simulink model "rx2"  (R2022b)
settings: Solver=FixedStepDiscrete  StartTime=0.0  StopTime=3.3E6  FixedStep=1  RelTol=1e-3  EnableMultiTasking=on
model workspace (MAT data in the model file):
  mwTaskManagerKernelLatency = 0
undefined symbols (not defined in the file or in its folder): Add, jsin, magnitude, rom_pilot_conj_tt, Shift
libraries: hdlsllib x3231, whdlutilities x525, simulink x260, whdlmod x112, whdledac x26, dsphdlmathfun2 x24, commchan3 x1
(part 30 of 59)

== system rx2/process4/decoder/rate recover/Subsystem ==
  start : Inport
  Compare To Constant : simulink/Logic and Bit Operations/Compare To Constant  relop===  const=valid_length  OutDataTypeStr=boolean
  Data Type Conversion : DataTypeConversion  OutDataTypeStr=boolean  SaturateOnIntegerOverflow=off  RndMeth=Floor
  Delay1 : Delay  InitialCondition=0
  Delay2 : Delay  DelayLength=1  InitialCondition=0
  Detect Fall Nonpositive : simulink/Logic and Bit Operations/Detect Fall Nonpositive  vinit=0  OutDataTypeStr=boolean
  HDL Counter1 : hdlsllib/Sources/HDL Counter  CountType=Count limited  CountInit=1  CountStep=1  CountMax=valid_length  CountFromType=Initial value  CountFrom=1  CountResetPort=off  CountLoadPort=off  CountEnbPort=on  CountDirPort=off  CountHitOutputPort=off  CountDataType=Unsigned  CountWordLen=16  CountFracLen=0  CountSampTime=1
  HDL Counter4 : hdlsllib/Sources/HDL Counter  CountType=Count limited  CountInit=0  CountStep=1  CountMax=1  CountFromType=Initial value  CountFrom=0  CountResetPort=on  CountLoadPort=off  CountEnbPort=on  CountDirPort=off  CountHitOutputPort=off  CountDataType=Unsigned  CountWordLen=8  CountFracLen=0  CountSampTime=1
  Logical Operator4 : Logic  AllPortsSameDT=off  OutDataTypeStr=boolean
  valid_out : Outport
  start_out : Outport  Port=2
  end_out : Outport  Port=3
  wires:
  Logical Operator4/1 -> end_out/1  "end_out"
  Delay2/1 -> valid_out/1, Logical Operator4/2  "valid_out"
  Delay1/1 -> start_out/1  "start_out"
  Data Type Conversion/1 -> HDL Counter1/1, Detect Fall Nonpositive/1, Delay2/1
  Detect Fall Nonpositive/1 -> Logical Operator4/1  "symbol_end"
  start/1 -> HDL Counter4/2, Delay1/1
  HDL Counter4/1 -> Data Type Conversion/1
  HDL Counter1/1 -> Compare To Constant/1  "count_1"
  Compare To Constant/1 -> HDL Counter4/1

== system rx2/process4/decoder/s-p/S-P ==
  data_in : Inport  OutDataTypeStr=fixdt(1,16,9)
  valid_in : Inport  Port=2  OutDataTypeStr=boolean
  Deserializer1D : hdlsllib/HDL Operations/Deserializer1D  Ratio=data_len  IdleCycles=8  InitialCondition=0  startIn=off  validIn=on  validOut=on  inputDataDimensions=-1  inputSampleTime=1  inputSignalType=real
  Rate Transition : RateTransition  OutPortSampleTimeOpt=Multiple of input port sample time  OutPortSampleTimeMultiple=1/72
  Rate Transition1 : RateTransition  OutPortSampleTimeOpt=Multiple of input port sample time  OutPortSampleTimeMultiple=1/72
  data_out : Outport  OutDataTypeStr=fixdt(1,16,9)
  valid_out : Outport  Port=2  OutDataTypeStr=boolean
  wires:
  valid_in/1 -> Deserializer1D/2  "valid_in"
  Rate Transition1/1 -> valid_out/1  "valid"
  Deserializer1D/2 -> Rate Transition1/1
  Rate Transition/1 -> data_out/1  "data"
  data_in/1 -> Deserializer1D/1
  Deserializer1D/1 -> Rate Transition/1

== system rx2/process4/decoder/s-p/S-P2 ==
  data_in : Inport  OutDataTypeStr=fixdt(1,16,9)
  valid_in : Inport  Port=2  OutDataTypeStr=boolean
  Deserializer1D : hdlsllib/HDL Operations/Deserializer1D  Ratio=data_len  IdleCycles=64  InitialCondition=0  startIn=off  validIn=on  validOut=on  inputDataDimensions=-1  inputSampleTime=1  inputSignalType=real
  Rate Transition : RateTransition  OutPortSampleTimeOpt=Multiple of input port sample time  OutPortSampleTimeMultiple=1/72
  Rate Transition1 : RateTransition  OutPortSampleTimeOpt=Multiple of input port sample time  OutPortSampleTimeMultiple=1/72
  data_out : Outport  OutDataTypeStr=fixdt(1,16,9)
  valid_out : Outport  Port=2  OutDataTypeStr=boolean
  wires:
  valid_in/1 -> Deserializer1D/2  "valid_in"
  Rate Transition1/1 -> valid_out/1  "valid"
  Deserializer1D/2 -> Rate Transition1/1
  Rate Transition/1 -> data_out/1  "data"
  data_in/1 -> Deserializer1D/1
  Deserializer1D/1 -> Rate Transition/1

== system rx2/process4/decoder/soft demodule/Subsystem ==
  start : Inport
  Compare To Constant : simulink/Logic and Bit Operations/Compare To Constant  relop===  const=valid_length  OutDataTypeStr=boolean
  Data Type Conversion : DataTypeConversion  OutDataTypeStr=boolean  SaturateOnIntegerOverflow=off  RndMeth=Floor
  Delay1 : Delay  InitialCondition=0
  Delay2 : Delay  DelayLength=1  InitialCondition=0
  Detect Fall Nonpositive : simulink/Logic and Bit Operations/Detect Fall Nonpositive  vinit=0  OutDataTypeStr=boolean
  HDL Counter1 : hdlsllib/Sources/HDL Counter  CountType=Count limited  CountInit=1  CountStep=1  CountMax=valid_length  CountFromType=Initial value  CountFrom=1  CountResetPort=off  CountLoadPort=off  CountEnbPort=on  CountDirPort=off  CountHitOutputPort=off  CountDataType=Unsigned  CountWordLen=16  CountFracLen=0  CountSampTime=1
  HDL Counter4 : hdlsllib/Sources/HDL Counter  CountType=Count limited  CountInit=0  CountStep=1  CountMax=1  CountFromType=Initial value  CountFrom=0  CountResetPort=on  CountLoadPort=off  CountEnbPort=on  CountDirPort=off  CountHitOutputPort=off  CountDataType=Unsigned  CountWordLen=8  CountFracLen=0  CountSampTime=1
  Logical Operator4 : Logic  AllPortsSameDT=off  OutDataTypeStr=boolean
  valid_out : Outport
  start_out : Outport  Port=2
  end_out : Outport  Port=3
  wires:
  Logical Operator4/1 -> end_out/1  "end_out"
  Delay2/1 -> valid_out/1, Logical Operator4/2  "valid_out"
  Delay1/1 -> start_out/1  "start_out"
  Data Type Conversion/1 -> HDL Counter1/1, Detect Fall Nonpositive/1, Delay2/1
  Detect Fall Nonpositive/1 -> Logical Operator4/1  "symbol_end"
  start/1 -> HDL Counter4/2, Delay1/1
  HDL Counter4/1 -> Data Type Conversion/1
  HDL Counter1/1 -> Compare To Constant/1  "count_1"
  Compare To Constant/1 -> HDL Counter4/1

== system rx2/process4/decoder/synchronization/data_synchronization1 ==
  port1 : Inport
  port2 : Inport  Port=2
  port1_ctrl : Inport  Port=3  OutDataTypeStr=Bus: samplecontrol
  port2_ctrl : Inport  Port=4  OutDataTypeStr=Bus: samplecontrol
  Bit Concat : hdlsllib/Logic and Bit Operations/Bit Concat  numInputs=2
  Compare To Constant10 : hdlsllib/Logic and Bit Operations/Compare To Constant  relop===  const=1  OutDataTypeStr=boolean
  Constant3 : Constant  OutDataTypeStr=fixdt(0,2,0)
  Data Type Conversion1 : DataTypeConversion  OutDataTypeStr=boolean  SaturateOnIntegerOverflow=off  RndMeth=Floor
  Delay1 : Delay  DelayLength=3  InitialCondition=0  SampleTime=1
  Delay{3..7,10..11} (7 alike) : Delay  DelayLength=1  InitialCondition=0
  Delay2 : Delay  DelayLength=3  InitialCondition=0  SampleTime=1
  Delay8 : Delay  DelayLength=3  InitialCondition=0
  Delay9 : Delay  DelayLength=3  InitialCondition=0
  Detect Rise Positive : simulink/Logic and Bit Operations/Detect Rise Positive  vinit=0  OutDataTypeStr=boolean
  Detect Rise Positive5 : hdlsllib/Logic and Bit Operations/Detect Rise Positive  vinit=0  OutDataTypeStr=boolean
  Ground3 : Ground
  Ground4 : Ground
  HDL Counter3 : hdlsllib/Sources/HDL Counter  CountType=Count limited  CountInit=0  CountStep=1  CountMax=2  CountFromType=Initial value  CountFrom=0  CountResetPort=on  CountLoadPort=off  CountEnbPort=on  CountDirPort=off  CountHitOutputPort=on  CountDataType=Unsigned  CountWordLen=2  CountFracLen=0  CountSampTime=1
  HDL Counter4 : hdlsllib/Sources/HDL Counter  CountType=Count limited  CountInit=0  CountStep=1  CountMax=2  CountFromType=Initial value  CountFrom=0  CountResetPort=on  CountLoadPort=off  CountEnbPort=on  CountDirPort=off  CountHitOutputPort=on  CountDataType=Unsigned  CountWordLen=2  CountFracLen=0  CountSampTime=1
  HDL Counter5 : hdlsllib/Sources/HDL Counter  CountType=Count limited  CountInit=0  CountStep=1  CountMax=1  CountFromType=Initial value  CountFrom=0  CountResetPort=off  CountLoadPort=off  CountEnbPort=on  CountDirPort=off  CountHitOutputPort=off  CountDataType=Unsigned  CountWordLen=1  CountFracLen=0  CountSampTime=1
  HDL FIFO : hdlsllib/HDL RAMs/HDL FIFO  fifo_size=792  mode=Classic  ratio=1  push_msg=Warning  pop_msg=Ignore  show_empty=on  show_full=on  show_num=on  LabelModeActiveChoice_Mode=Classic  rst_port=off
  Logical Operator : Logic  Operator=OR  AllPortsSameDT=off  OutDataTypeStr=boolean
  Logical Operator8 : Logic  Operator=OR  AllPortsSameDT=off  OutDataTypeStr=boolean
  Logical Operator9 : Logic  Operator=OR  AllPortsSameDT=off  OutDataTypeStr=boolean
  Multiport Switch{1..5} (5 alike) : MultiPortSwitch  Inputs=2  DiagnosticForDefault=None  SaturateOnIntegerOverflow=off  InputSameDT=off
  Sample Control Bus Selector : whdlutilities/Sample Control Bus Selector  OutputSignals=start,end,valid
  Sample Control Bus Selector1 : whdlutilities/Sample Control Bus Selector  OutputSignals=start,end,valid
  Simple Dual Port RAM : hdlsllib/HDL RAMs/Simple Dual Port RAM  ram_size=2
  Switch5 : Switch  Criteria=u2 ~= 0  SaturateOnIntegerOverflow=off  InputSameDT=off
  Switch6 : Switch  Criteria=u2 ~= 0  SaturateOnIntegerOverflow=off  InputSameDT=off
  Terminator{,1..3} (4 alike) : Terminator
  port1_syn : Outport  VectorParamsAs1DForOutWhenUnconnected=off
  port2_syn : Outport  Port=2  VectorParamsAs1DForOutWhenUnconnected=off
  valid_syn : Outport  Port=3  OutDataTypeStr=boolean  VectorParamsAs1DForOutWhenUnconnected=off
  start_syn : Outport  Port=4  OutDataTypeStr=boolean  VectorParamsAs1DForOutWhenUnconnected=off
  wires:
  port1_ctrl/1 -> Sample Control Bus Selector/1
  port2_ctrl/1 -> Sample Control Bus Selector1/1
  Sample Control Bus Selector/1 -> Logical Operator/1
  Sample Control Bus Selector1/1 -> Logical Operator/2
  Sample Control Bus Selector/2 -> Logical Operator8/1
  Delay7/1 -> HDL Counter4/1
  HDL Counter4/2 -> Delay7/1
  Compare To Constant10/1 -> Detect Rise Positive5/1
  Logical Operator8/1 -> HDL Counter3/2
  HDL Counter3/2 -> Logical Operator9/2, Delay6/1
  HDL Counter3/1 -> Terminator2/1
  Delay6/1 -> HDL Counter3/1
  Logical Operator/1 -> HDL Counter4/2
  Detect Rise Positive5/1 -> Logical Operator9/1
  HDL Counter4/1 -> Compare To Constant10/1
  HDL Counter5/1 -> Data Type Conversion1/1
  Logical Operator9/1 -> HDL Counter5/1, Simple Dual Port RAM/3
  Bit Concat/1 -> Simple Dual Port RAM/1
  Constant3/1 -> Simple Dual Port RAM/4, Simple Dual Port RAM/2
  Data Type Conversion1/1 -> Delay3/1
  Sample Control Bus Selector1/2 -> Logical Operator8/2
  Simple Dual Port RAM/1 -> [number]
  port1/1 -> Delay1/1
  port2/1 -> Delay2/1
  Multiport Switch1/1 -> HDL FIFO/2
  HDL FIFO/1 -> Multiport Switch5/3, Multiport Switch4/2
  HDL FIFO/3 -> Terminator/1
  Multiport Switch3/1 -> HDL FIFO/1
  Multiport Switch2/1 -> Delay11/1, HDL FIFO/3
  [number] -> Multiport Switch2/1, Multiport Switch1/1, Multiport Switch3/1
  Sample Control Bus Selector/3 -> Delay9/1, Bit Concat/2
  Sample Control Bus Selector1/3 -> Delay8/1, Bit Concat/1
  Delay2/1 -> [P2], Multiport Switch3/3
  Delay3/1 -> [number_valid]
  Delay8/1 -> Multiport Switch2/2, Multiport Switch1/3
  Delay9/1 -> Multiport Switch2/3, Multiport Switch1/2
  HDL FIFO/2 -> Terminator1/1
  HDL FIFO/4 -> Terminator3/1
  [number] -> Delay4/1
  Delay4/1 -> Multiport Switch5/1, Multiport Switch4/1
  Delay1/1 -> [P1], Multiport Switch3/2
  [P1] -> Delay5/1
  [P2] -> Delay10/1
  Delay10/1 -> Multiport Switch5/2
  Delay5/1 -> Multiport Switch4/3
  Ground4/1 -> Switch6/3
  Switch5/1 -> port1_syn/1  "port1_syn"
  Switch6/1 -> port2_syn/1  "port2_syn"
  Ground3/1 -> Switch5/3
  Multiport Switch4/1 -> Switch5/1
  Multiport Switch5/1 -> Switch6/1
  Delay11/1 -> Switch5/2, Switch6/2, Detect Rise Positive/1, valid_syn/1
  Detect Rise Positive/1 -> start_syn/1

== system rx2/process4/decoder/synchronization/data_synchronization2 ==
  port1 : Inport
  port2 : Inport  Port=2
  port1_ctrl : Inport  Port=3  OutDataTypeStr=Bus: samplecontrol
  port2_ctrl : Inport  Port=4  OutDataTypeStr=Bus: samplecontrol
  Bit Concat : hdlsllib/Logic and Bit Operations/Bit Concat  numInputs=2
  Compare To Constant10 : hdlsllib/Logic and Bit Operations/Compare To Constant  relop===  const=1  OutDataTypeStr=boolean
  Constant3 : Constant  OutDataTypeStr=fixdt(0,2,0)
  Data Type Conversion1 : DataTypeConversion  OutDataTypeStr=boolean  SaturateOnIntegerOverflow=off  RndMeth=Floor
  Delay1 : Delay  DelayLength=3  InitialCondition=0  SampleTime=1
  Delay{3..7,10..11} (7 alike) : Delay  DelayLength=1  InitialCondition=0
  Delay2 : Delay  DelayLength=3  InitialCondition=0  SampleTime=1
  Delay8 : Delay  DelayLength=3  InitialCondition=0
  Delay9 : Delay  DelayLength=3  InitialCondition=0
  Detect Rise Positive : simulink/Logic and Bit Operations/Detect Rise Positive  vinit=0  OutDataTypeStr=boolean
  Detect Rise Positive5 : hdlsllib/Logic and Bit Operations/Detect Rise Positive  vinit=0  OutDataTypeStr=boolean
  Ground3 : Ground
  Ground4 : Ground
  HDL Counter3 : hdlsllib/Sources/HDL Counter  CountType=Count limited  CountInit=0  CountStep=1  CountMax=2  CountFromType=Initial value  CountFrom=0  CountResetPort=on  CountLoadPort=off  CountEnbPort=on  CountDirPort=off  CountHitOutputPort=on  CountDataType=Unsigned  CountWordLen=2  CountFracLen=0  CountSampTime=1
  HDL Counter4 : hdlsllib/Sources/HDL Counter  CountType=Count limited  CountInit=0  CountStep=1  CountMax=2  CountFromType=Initial value  CountFrom=0  CountResetPort=on  CountLoadPort=off  CountEnbPort=on  CountDirPort=off  CountHitOutputPort=on  CountDataType=Unsigned  CountWordLen=2  CountFracLen=0  CountSampTime=1
  HDL Counter5 : hdlsllib/Sources/HDL Counter  CountType=Count limited  CountInit=0  CountStep=1  CountMax=1  CountFromType=Initial value  CountFrom=0  CountResetPort=off  CountLoadPort=off  CountEnbPort=on  CountDirPort=off  CountHitOutputPort=off  CountDataType=Unsigned  CountWordLen=1  CountFracLen=0  CountSampTime=1
  HDL FIFO : hdlsllib/HDL RAMs/HDL FIFO  fifo_size=792  mode=Classic  ratio=1  push_msg=Warning  pop_msg=Ignore  show_empty=on  show_full=on  show_num=on  LabelModeActiveChoice_Mode=Classic  rst_port=off
  Logical Operator : Logic  Operator=OR  AllPortsSameDT=off  OutDataTypeStr=boolean
  Logical Operator8 : Logic  Operator=OR  AllPortsSameDT=off  OutDataTypeStr=boolean
  Logical Operator9 : Logic  Operator=OR  AllPortsSameDT=off  OutDataTypeStr=boolean
  Multiport Switch{1..5} (5 alike) : MultiPortSwitch  Inputs=2  DiagnosticForDefault=None  SaturateOnIntegerOverflow=off  InputSameDT=off
  Sample Control Bus Selector : whdlutilities/Sample Control Bus Selector  OutputSignals=start,end,valid
  Sample Control Bus Selector1 : whdlutilities/Sample Control Bus Selector  OutputSignals=start,end,valid
  Simple Dual Port RAM : hdlsllib/HDL RAMs/Simple Dual Port RAM  ram_size=2
  Switch5 : Switch  Criteria=u2 ~= 0  SaturateOnIntegerOverflow=off  InputSameDT=off
  Switch6 : Switch  Criteria=u2 ~= 0  SaturateOnIntegerOverflow=off  InputSameDT=off
  Terminator{,1..3} (4 alike) : Terminator
  port1_syn : Outport  VectorParamsAs1DForOutWhenUnconnected=off
  port2_syn : Outport  Port=2  VectorParamsAs1DForOutWhenUnconnected=off
  valid_syn : Outport  Port=3  OutDataTypeStr=boolean  VectorParamsAs1DForOutWhenUnconnected=off
  start_syn : Outport  Port=4  OutDataTypeStr=boolean  VectorParamsAs1DForOutWhenUnconnected=off
  wires:
  port1_ctrl/1 -> Sample Control Bus Selector/1
  port2_ctrl/1 -> Sample Control Bus Selector1/1
  Sample Control Bus Selector/1 -> Logical Operator/1
  Sample Control Bus Selector1/1 -> Logical Operator/2
  Sample Control Bus Selector/2 -> Logical Operator8/1
  Delay7/1 -> HDL Counter4/1
  HDL Counter4/2 -> Delay7/1
  Compare To Constant10/1 -> Detect Rise Positive5/1
  Logical Operator8/1 -> HDL Counter3/2
  HDL Counter3/2 -> Logical Operator9/2, Delay6/1
  HDL Counter3/1 -> Terminator2/1
  Delay6/1 -> HDL Counter3/1
  Logical Operator/1 -> HDL Counter4/2
  Detect Rise Positive5/1 -> Logical Operator9/1
  HDL Counter4/1 -> Compare To Constant10/1
  HDL Counter5/1 -> Data Type Conversion1/1
  Logical Operator9/1 -> HDL Counter5/1, Simple Dual Port RAM/3
  Bit Concat/1 -> Simple Dual Port RAM/1
  Constant3/1 -> Simple Dual Port RAM/4, Simple Dual Port RAM/2
  Data Type Conversion1/1 -> Delay3/1
  Sample Control Bus Selector1/2 -> Logical Operator8/2
  Simple Dual Port RAM/1 -> [number]
  port1/1 -> Delay1/1
  port2/1 -> Delay2/1
  Multiport Switch1/1 -> HDL FIFO/2
  HDL FIFO/1 -> Multiport Switch5/3, Multiport Switch4/2
  HDL FIFO/3 -> Terminator/1
  Multiport Switch3/1 -> HDL FIFO/1
  Multiport Switch2/1 -> HDL FIFO/3, Delay11/1
  [number] -> Multiport Switch2/1, Multiport Switch1/1, Multiport Switch3/1
  Sample Control Bus Selector/3 -> Delay9/1, Bit Concat/2
  Sample Control Bus Selector1/3 -> Delay8/1, Bit Concat/1
  Delay2/1 -> [P2], Multiport Switch3/3
  Delay3/1 -> [number_valid]
  Delay8/1 -> Multiport Switch2/2, Multiport Switch1/3
  Delay9/1 -> Multiport Switch2/3, Multiport Switch1/2
  HDL FIFO/2 -> Terminator1/1
  HDL FIFO/4 -> Terminator3/1
  [number] -> Delay4/1
  Delay4/1 -> Multiport Switch5/1, Multiport Switch4/1
  Delay1/1 -> [P1], Multiport Switch3/2
  [P1] -> Delay5/1
  [P2] -> Delay10/1
  Delay10/1 -> Multiport Switch5/2
  Delay5/1 -> Multiport Switch4/3
  Ground4/1 -> Switch6/3
  Switch5/1 -> port1_syn/1  "port1_syn"
  Switch6/1 -> port2_syn/1  "port2_syn"
  Ground3/1 -> Switch5/3
  Multiport Switch4/1 -> Switch5/1
  Multiport Switch5/1 -> Switch6/1
  Delay11/1 -> Switch5/2, Switch6/2, Detect Rise Positive/1, valid_syn/1
  Detect Rise Positive/1 -> start_syn/1

== system rx2/process4/decoder/synchronization/data_synchronization3 ==
  port1 : Inport
  port2 : Inport  Port=2
  port1_ctrl : Inport  Port=3  OutDataTypeStr=Bus: samplecontrol
  port2_ctrl : Inport  Port=4  OutDataTypeStr=Bus: samplecontrol
  Bit Concat : hdlsllib/Logic and Bit Operations/Bit Concat  numInputs=2
  Compare To Constant10 : hdlsllib/Logic and Bit Operations/Compare To Constant  relop===  const=1  OutDataTypeStr=boolean
  Constant3 : Constant  OutDataTypeStr=fixdt(0,2,0)
  Data Type Conversion1 : DataTypeConversion  OutDataTypeStr=boolean  SaturateOnIntegerOverflow=off  RndMeth=Floor
  Delay1 : Delay  DelayLength=3  InitialCondition=0  SampleTime=1
  Delay{3..7,10..11} (7 alike) : Delay  DelayLength=1  InitialCondition=0
  Delay2 : Delay  DelayLength=3  InitialCondition=0  SampleTime=1
  Delay8 : Delay  DelayLength=3  InitialCondition=0
  Delay9 : Delay  DelayLength=3  InitialCondition=0
  Detect Rise Positive : simulink/Logic and Bit Operations/Detect Rise Positive  vinit=0  OutDataTypeStr=boolean
  Detect Rise Positive5 : hdlsllib/Logic and Bit Operations/Detect Rise Positive  vinit=0  OutDataTypeStr=boolean
  Ground3 : Ground
  Ground4 : Ground
  HDL Counter3 : hdlsllib/Sources/HDL Counter  CountType=Count limited  CountInit=0  CountStep=1  CountMax=2  CountFromType=Initial value  CountFrom=0  CountResetPort=on  CountLoadPort=off  CountEnbPort=on  CountDirPort=off  CountHitOutputPort=on  CountDataType=Unsigned  CountWordLen=2  CountFracLen=0  CountSampTime=1
  HDL Counter4 : hdlsllib/Sources/HDL Counter  CountType=Count limited  CountInit=0  CountStep=1  CountMax=2  CountFromType=Initial value  CountFrom=0  CountResetPort=on  CountLoadPort=off  CountEnbPort=on  CountDirPort=off  CountHitOutputPort=on  CountDataType=Unsigned  CountWordLen=2  CountFracLen=0  CountSampTime=1
  HDL Counter5 : hdlsllib/Sources/HDL Counter  CountType=Count limited  CountInit=0  CountStep=1  CountMax=1  CountFromType=Initial value  CountFrom=0  CountResetPort=off  CountLoadPort=off  CountEnbPort=on  CountDirPort=off  CountHitOutputPort=off  CountDataType=Unsigned  CountWordLen=1  CountFracLen=0  CountSampTime=1
  HDL FIFO : hdlsllib/HDL RAMs/HDL FIFO  fifo_size=792  mode=Classic  ratio=1  push_msg=Warning  pop_msg=Ignore  show_empty=on  show_full=on  show_num=on  LabelModeActiveChoice_Mode=Classic  rst_port=off
  Logical Operator : Logic  Operator=OR  AllPortsSameDT=off  OutDataTypeStr=boolean
  Logical Operator8 : Logic  Operator=OR  AllPortsSameDT=off  OutDataTypeStr=boolean
  Logical Operator9 : Logic  Operator=OR  AllPortsSameDT=off  OutDataTypeStr=boolean
  Multiport Switch{1..5} (5 alike) : MultiPortSwitch  Inputs=2  DiagnosticForDefault=None  SaturateOnIntegerOverflow=off  InputSameDT=off
  Sample Control Bus Selector : whdlutilities/Sample Control Bus Selector  OutputSignals=start,end,valid
  Sample Control Bus Selector1 : whdlutilities/Sample Control Bus Selector  OutputSignals=start,end,valid
  Simple Dual Port RAM : hdlsllib/HDL RAMs/Simple Dual Port RAM  ram_size=2
  Switch5 : Switch  Criteria=u2 ~= 0  SaturateOnIntegerOverflow=off  InputSameDT=off
  Switch6 : Switch  Criteria=u2 ~= 0  SaturateOnIntegerOverflow=off  InputSameDT=off
  Terminator{,1..3} (4 alike) : Terminator
  port1_syn : Outport  VectorParamsAs1DForOutWhenUnconnected=off
  port2_syn : Outport  Port=2  VectorParamsAs1DForOutWhenUnconnected=off
  valid_syn : Outport  Port=3  OutDataTypeStr=boolean  VectorParamsAs1DForOutWhenUnconnected=off
  start_syn : Outport  Port=4  OutDataTypeStr=boolean  VectorParamsAs1DForOutWhenUnconnected=off
  wires:
  port1_ctrl/1 -> Sample Control Bus Selector/1
  port2_ctrl/1 -> Sample Control Bus Selector1/1
  Sample Control Bus Selector/1 -> Logical Operator/1
  Sample Control Bus Selector1/1 -> Logical Operator/2
  Sample Control Bus Selector/2 -> Logical Operator8/1
  Delay7/1 -> HDL Counter4/1
  HDL Counter4/2 -> Delay7/1
  Compare To Constant10/1 -> Detect Rise Positive5/1
  Logical Operator8/1 -> HDL Counter3/2
  HDL Counter3/2 -> Logical Operator9/2, Delay6/1
  HDL Counter3/1 -> Terminator2/1
  Delay6/1 -> HDL Counter3/1
  Logical Operator/1 -> HDL Counter4/2
  Detect Rise Positive5/1 -> Logical Operator9/1
  HDL Counter4/1 -> Compare To Constant10/1
  HDL Counter5/1 -> Data Type Conversion1/1
  Logical Operator9/1 -> HDL Counter5/1, Simple Dual Port RAM/3
  Bit Concat/1 -> Simple Dual Port RAM/1
  Constant3/1 -> Simple Dual Port RAM/4, Simple Dual Port RAM/2
  Data Type Conversion1/1 -> Delay3/1
  Sample Control Bus Selector1/2 -> Logical Operator8/2
  Simple Dual Port RAM/1 -> [number]
  port1/1 -> Delay1/1
  port2/1 -> Delay2/1
  Multiport Switch1/1 -> HDL FIFO/2
  HDL FIFO/1 -> Multiport Switch5/3, Multiport Switch4/2
  HDL FIFO/3 -> Terminator/1
  Multiport Switch3/1 -> HDL FIFO/1
  Multiport Switch2/1 -> HDL FIFO/3, Delay11/1
  [number] -> Multiport Switch2/1, Multiport Switch1/1, Multiport Switch3/1
  Sample Control Bus Selector/3 -> Delay9/1, Bit Concat/2
  Sample Control Bus Selector1/3 -> Delay8/1, Bit Concat/1
  Delay2/1 -> [P2], Multiport Switch3/3
  Delay3/1 -> [number_valid]
  Delay8/1 -> Multiport Switch2/2, Multiport Switch1/3
  Delay9/1 -> Multiport Switch2/3, Multiport Switch1/2
  HDL FIFO/2 -> Terminator1/1
  HDL FIFO/4 -> Terminator3/1
  [number] -> Delay4/1
  Delay4/1 -> Multiport Switch5/1, Multiport Switch4/1
  Delay1/1 -> [P1], Multiport Switch3/2
  [P1] -> Delay5/1
  [P2] -> Delay10/1
  Delay10/1 -> Multiport Switch5/2
  Delay5/1 -> Multiport Switch4/3
  Ground4/1 -> Switch6/3
  Switch5/1 -> port1_syn/1  "port1_syn"
  Switch6/1 -> port2_syn/1  "port2_syn"
  Ground3/1 -> Switch5/3
  Multiport Switch4/1 -> Switch5/1
  Multiport Switch5/1 -> Switch6/1
  Delay11/1 -> Switch5/2, Switch6/2, Detect Rise Positive/1, valid_syn/1
  Detect Rise Positive/1 -> start_syn/1

== system rx2/process4/decoder/synchronization/data_synchronization4 ==
  port1 : Inport
  port2 : Inport  Port=2
  port1_ctrl : Inport  Port=3  OutDataTypeStr=Bus: samplecontrol
  port2_ctrl : Inport  Port=4  OutDataTypeStr=Bus: samplecontrol
  Bit Concat : hdlsllib/Logic and Bit Operations/Bit Concat  numInputs=2
  Compare To Constant10 : hdlsllib/Logic and Bit Operations/Compare To Constant  relop===  const=1  OutDataTypeStr=boolean
  Constant3 : Constant  OutDataTypeStr=fixdt(0,2,0)
  Data Type Conversion1 : DataTypeConversion  OutDataTypeStr=boolean  SaturateOnIntegerOverflow=off  RndMeth=Floor
  Delay1 : Delay  DelayLength=3  InitialCondition=0  SampleTime=1
  Delay{3..7,10..11} (7 alike) : Delay  DelayLength=1  InitialCondition=0
  Delay2 : Delay  DelayLength=3  InitialCondition=0  SampleTime=1
  Delay8 : Delay  DelayLength=3  InitialCondition=0
  Delay9 : Delay  DelayLength=3  InitialCondition=0
  Detect Rise Positive : simulink/Logic and Bit Operations/Detect Rise Positive  vinit=0  OutDataTypeStr=boolean
  Detect Rise Positive5 : hdlsllib/Logic and Bit Operations/Detect Rise Positive  vinit=0  OutDataTypeStr=boolean
  Ground3 : Ground
  Ground4 : Ground
  HDL Counter3 : hdlsllib/Sources/HDL Counter  CountType=Count limited  CountInit=0  CountStep=1  CountMax=2  CountFromType=Initial value  CountFrom=0  CountResetPort=on  CountLoadPort=off  CountEnbPort=on  CountDirPort=off  CountHitOutputPort=on  CountDataType=Unsigned  CountWordLen=2  CountFracLen=0  CountSampTime=1
  HDL Counter4 : hdlsllib/Sources/HDL Counter  CountType=Count limited  CountInit=0  CountStep=1  CountMax=2  CountFromType=Initial value  CountFrom=0  CountResetPort=on  CountLoadPort=off  CountEnbPort=on  CountDirPort=off  CountHitOutputPort=on  CountDataType=Unsigned  CountWordLen=2  CountFracLen=0  CountSampTime=1
  HDL Counter5 : hdlsllib/Sources/HDL Counter  CountType=Count limited  CountInit=0  CountStep=1  CountMax=1  CountFromType=Initial value  CountFrom=0  CountResetPort=off  CountLoadPort=off  CountEnbPort=on  CountDirPort=off  CountHitOutputPort=off  CountDataType=Unsigned  CountWordLen=1  CountFracLen=0  CountSampTime=1
  HDL FIFO : hdlsllib/HDL RAMs/HDL FIFO  fifo_size=792  mode=Classic  ratio=1  push_msg=Warning  pop_msg=Ignore  show_empty=on  show_full=on  show_num=on  LabelModeActiveChoice_Mode=Classic  rst_port=off
  Logical Operator : Logic  Operator=OR  AllPortsSameDT=off  OutDataTypeStr=boolean
  Logical Operator8 : Logic  Operator=OR  AllPortsSameDT=off  OutDataTypeStr=boolean
  Logical Operator9 : Logic  Operator=OR  AllPortsSameDT=off  OutDataTypeStr=boolean
  Multiport Switch{1..5} (5 alike) : MultiPortSwitch  Inputs=2  DiagnosticForDefault=None  SaturateOnIntegerOverflow=off  InputSameDT=off
  Sample Control Bus Selector : whdlutilities/Sample Control Bus Selector  OutputSignals=start,end,valid
  Sample Control Bus Selector1 : whdlutilities/Sample Control Bus Selector  OutputSignals=start,end,valid
  Simple Dual Port RAM : hdlsllib/HDL RAMs/Simple Dual Port RAM  ram_size=2
  Switch5 : Switch  Criteria=u2 ~= 0  SaturateOnIntegerOverflow=off  InputSameDT=off
  Switch6 : Switch  Criteria=u2 ~= 0  SaturateOnIntegerOverflow=off  InputSameDT=off
  Terminator{,1..3} (4 alike) : Terminator
  port1_syn : Outport  VectorParamsAs1DForOutWhenUnconnected=off
  port2_syn : Outport  Port=2  VectorParamsAs1DForOutWhenUnconnected=off
  valid_syn : Outport  Port=3  OutDataTypeStr=boolean  VectorParamsAs1DForOutWhenUnconnected=off
  start_syn : Outport  Port=4  OutDataTypeStr=boolean  VectorParamsAs1DForOutWhenUnconnected=off
  wires:
  port1_ctrl/1 -> Sample Control Bus Selector/1
  port2_ctrl/1 -> Sample Control Bus Selector1/1
  Sample Control Bus Selector/1 -> Logical Operator/1
  Sample Control Bus Selector1/1 -> Logical Operator/2
  Sample Control Bus Selector/2 -> Logical Operator8/1
  Delay7/1 -> HDL Counter4/1
  HDL Counter4/2 -> Delay7/1
  Compare To Constant10/1 -> Detect Rise Positive5/1
  Logical Operator8/1 -> HDL Counter3/2
  HDL Counter3/2 -> Logical Operator9/2, Delay6/1
  HDL Counter3/1 -> Terminator2/1
  Delay6/1 -> HDL Counter3/1
  Logical Operator/1 -> HDL Counter4/2
  Detect Rise Positive5/1 -> Logical Operator9/1
  HDL Counter4/1 -> Compare To Constant10/1
  HDL Counter5/1 -> Data Type Conversion1/1
  Logical Operator9/1 -> HDL Counter5/1, Simple Dual Port RAM/3
  Bit Concat/1 -> Simple Dual Port RAM/1
  Constant3/1 -> Simple Dual Port RAM/4, Simple Dual Port RAM/2
  Data Type Conversion1/1 -> Delay3/1
  Sample Control Bus Selector1/2 -> Logical Operator8/2
  Simple Dual Port RAM/1 -> [number]
  port1/1 -> Delay1/1
  port2/1 -> Delay2/1
  Multiport Switch1/1 -> HDL FIFO/2
  HDL FIFO/1 -> Multiport Switch5/3, Multiport Switch4/2
  HDL FIFO/3 -> Terminator/1
  Multiport Switch3/1 -> HDL FIFO/1
  Multiport Switch2/1 -> HDL FIFO/3, Delay11/1
  [number] -> Multiport Switch2/1, Multiport Switch1/1, Multiport Switch3/1
  Sample Control Bus Selector/3 -> Delay9/1, Bit Concat/2
  Sample Control Bus Selector1/3 -> Delay8/1, Bit Concat/1
  Delay2/1 -> [P2], Multiport Switch3/3
  Delay3/1 -> [number_valid]
  Delay8/1 -> Multiport Switch2/2, Multiport Switch1/3
  Delay9/1 -> Multiport Switch2/3, Multiport Switch1/2
  HDL FIFO/2 -> Terminator1/1
  HDL FIFO/4 -> Terminator3/1
  [number] -> Delay4/1
  Delay4/1 -> Multiport Switch5/1, Multiport Switch4/1
  Delay1/1 -> [P1], Multiport Switch3/2
  [P1] -> Delay5/1
  [P2] -> Delay10/1
  Delay10/1 -> Multiport Switch5/2
  Delay5/1 -> Multiport Switch4/3
  Ground4/1 -> Switch6/3
  Switch5/1 -> port1_syn/1  "port1_syn"
  Switch6/1 -> port2_syn/1  "port2_syn"
  Ground3/1 -> Switch5/3
  Multiport Switch4/1 -> Switch5/1
  Multiport Switch5/1 -> Switch6/1
  Delay11/1 -> Switch5/2, Switch6/2, Detect Rise Positive/1, valid_syn/1
  Detect Rise Positive/1 -> start_syn/1

== system rx2/process4/decoder/synchronization/data_synchronization5 ==
  port1 : Inport
  port2 : Inport  Port=2
  port1_ctrl : Inport  Port=3  OutDataTypeStr=Bus: samplecontrol
  port2_ctrl : Inport  Port=4  OutDataTypeStr=Bus: samplecontrol
  Bit Concat : hdlsllib/Logic and Bit Operations/Bit Concat  numInputs=2
  Compare To Constant10 : hdlsllib/Logic and Bit Operations/Compare To Constant  relop===  const=1  OutDataTypeStr=boolean
  Constant3 : Constant  OutDataTypeStr=fixdt(0,2,0)
  Data Type Conversion1 : DataTypeConversion  OutDataTypeStr=boolean  SaturateOnIntegerOverflow=off  RndMeth=Floor
  Delay1 : Delay  DelayLength=3  InitialCondition=0  SampleTime=1
  Delay{3..7,10..11} (7 alike) : Delay  DelayLength=1  InitialCondition=0
  Delay2 : Delay  DelayLength=3  InitialCondition=0  SampleTime=1
  Delay8 : Delay  DelayLength=3  InitialCondition=0
  Delay9 : Delay  DelayLength=3  InitialCondition=0
  Detect Rise Positive : simulink/Logic and Bit Operations/Detect Rise Positive  vinit=0  OutDataTypeStr=boolean
  Detect Rise Positive5 : hdlsllib/Logic and Bit Operations/Detect Rise Positive  vinit=0  OutDataTypeStr=boolean
  Ground3 : Ground
  Ground4 : Ground
  HDL Counter3 : hdlsllib/Sources/HDL Counter  CountType=Count limited  CountInit=0  CountStep=1  CountMax=2  CountFromType=Initial value  CountFrom=0  CountResetPort=on  CountLoadPort=off  CountEnbPort=on  CountDirPort=off  CountHitOutputPort=on  CountDataType=Unsigned  CountWordLen=2  CountFracLen=0  CountSampTime=1
  HDL Counter4 : hdlsllib/Sources/HDL Counter  CountType=Count limited  CountInit=0  CountStep=1  CountMax=2  CountFromType=Initial value  CountFrom=0  CountResetPort=on  CountLoadPort=off  CountEnbPort=on  CountDirPort=off  CountHitOutputPort=on  CountDataType=Unsigned  CountWordLen=2  CountFracLen=0  CountSampTime=1
  HDL Counter5 : hdlsllib/Sources/HDL Counter  CountType=Count limited  CountInit=0  CountStep=1  CountMax=1  CountFromType=Initial value  CountFrom=0  CountResetPort=off  CountLoadPort=off  CountEnbPort=on  CountDirPort=off  CountHitOutputPort=off  CountDataType=Unsigned  CountWordLen=1  CountFracLen=0  CountSampTime=1
  HDL FIFO : hdlsllib/HDL RAMs/HDL FIFO  fifo_size=792  mode=Classic  ratio=1  push_msg=Warning  pop_msg=Ignore  show_empty=on  show_full=on  show_num=on  LabelModeActiveChoice_Mode=Classic  rst_port=off
  Logical Operator : Logic  Operator=OR  AllPortsSameDT=off  OutDataTypeStr=boolean
  Logical Operator8 : Logic  Operator=OR  AllPortsSameDT=off  OutDataTypeStr=boolean
  Logical Operator9 : Logic  Operator=OR  AllPortsSameDT=off  OutDataTypeStr=boolean
  Multiport Switch{1..5} (5 alike) : MultiPortSwitch  Inputs=2  DiagnosticForDefault=None  SaturateOnIntegerOverflow=off  InputSameDT=off
  Sample Control Bus Selector : whdlutilities/Sample Control Bus Selector  OutputSignals=start,end,valid
  Sample Control Bus Selector1 : whdlutilities/Sample Control Bus Selector  OutputSignals=start,end,valid
  Simple Dual Port RAM : hdlsllib/HDL RAMs/Simple Dual Port RAM  ram_size=2
  Switch5 : Switch  Criteria=u2 ~= 0  SaturateOnIntegerOverflow=off  InputSameDT=off
  Switch6 : Switch  Criteria=u2 ~= 0  SaturateOnIntegerOverflow=off  InputSameDT=off
  Terminator{,1..3} (4 alike) : Terminator
  port1_syn : Outport  VectorParamsAs1DForOutWhenUnconnected=off
  port2_syn : Outport  Port=2  VectorParamsAs1DForOutWhenUnconnected=off
  valid_syn : Outport  Port=3  OutDataTypeStr=boolean  VectorParamsAs1DForOutWhenUnconnected=off
  start_syn : Outport  Port=4  OutDataTypeStr=boolean  VectorParamsAs1DForOutWhenUnconnected=off
  wires:
  port1_ctrl/1 -> Sample Control Bus Selector/1
  port2_ctrl/1 -> Sample Control Bus Selector1/1
  Sample Control Bus Selector/1 -> Logical Operator/1
  Sample Control Bus Selector1/1 -> Logical Operator/2
  Sample Control Bus Selector/2 -> Logical Operator8/1
  Delay7/1 -> HDL Counter4/1
  HDL Counter4/2 -> Delay7/1
  Compare To Constant10/1 -> Detect Rise Positive5/1
  Logical Operator8/1 -> HDL Counter3/2
  HDL Counter3/2 -> Logical Operator9/2, Delay6/1
  HDL Counter3/1 -> Terminator2/1
  Delay6/1 -> HDL Counter3/1
  Logical Operator/1 -> HDL Counter4/2
  Detect Rise Positive5/1 -> Logical Operator9/1
  HDL Counter4/1 -> Compare To Constant10/1
  HDL Counter5/1 -> Data Type Conversion1/1
  Logical Operator9/1 -> HDL Counter5/1, Simple Dual Port RAM/3
  Bit Concat/1 -> Simple Dual Port RAM/1
  Constant3/1 -> Simple Dual Port RAM/4, Simple Dual Port RAM/2
  Data Type Conversion1/1 -> Delay3/1
  Sample Control Bus Selector1/2 -> Logical Operator8/2
  Simple Dual Port RAM/1 -> [number]
  port1/1 -> Delay1/1
  port2/1 -> Delay2/1
  Multiport Switch1/1 -> HDL FIFO/2
  HDL FIFO/1 -> Multiport Switch5/3, Multiport Switch4/2
  HDL FIFO/3 -> Terminator/1
  Multiport Switch3/1 -> HDL FIFO/1
  Multiport Switch2/1 -> HDL FIFO/3, Delay11/1
  [number] -> Multiport Switch2/1, Multiport Switch1/1, Multiport Switch3/1
  Sample Control Bus Selector/3 -> Delay9/1, Bit Concat/2
  Sample Control Bus Selector1/3 -> Delay8/1, Bit Concat/1
  Delay2/1 -> [P2], Multiport Switch3/3
  Delay3/1 -> [number_valid]
  Delay8/1 -> Multiport Switch2/2, Multiport Switch1/3
  Delay9/1 -> Multiport Switch2/3, Multiport Switch1/2
  HDL FIFO/2 -> Terminator1/1
  HDL FIFO/4 -> Terminator3/1
  [number] -> Delay4/1
  Delay4/1 -> Multiport Switch5/1, Multiport Switch4/1
  Delay1/1 -> [P1], Multiport Switch3/2
  [P1] -> Delay5/1
  [P2] -> Delay10/1
  Delay10/1 -> Multiport Switch5/2
  Delay5/1 -> Multiport Switch4/3
  Ground4/1 -> Switch6/3
  Switch5/1 -> port1_syn/1  "port1_syn"
  Switch6/1 -> port2_syn/1  "port2_syn"
  Ground3/1 -> Switch5/3
  Multiport Switch4/1 -> Switch5/1
  Multiport Switch5/1 -> Switch6/1
  Delay11/1 -> Switch5/2, Switch6/2, Detect Rise Positive/1, valid_syn/1
  Detect Rise Positive/1 -> start_syn/1

== system rx2/process4/decoder/synchronization/data_synchronization6 ==
  port1 : Inport
  port2 : Inport  Port=2
  port1_ctrl : Inport  Port=3  OutDataTypeStr=Bus: samplecontrol
  port2_ctrl : Inport  Port=4  OutDataTypeStr=Bus: samplecontrol
  Bit Concat : hdlsllib/Logic and Bit Operations/Bit Concat  numInputs=2
  Compare To Constant10 : hdlsllib/Logic and Bit Operations/Compare To Constant  relop===  const=1  OutDataTypeStr=boolean
  Constant3 : Constant  OutDataTypeStr=fixdt(0,2,0)
  Data Type Conversion1 : DataTypeConversion  OutDataTypeStr=boolean  SaturateOnIntegerOverflow=off  RndMeth=Floor
  Delay1 : Delay  DelayLength=3  InitialCondition=0  SampleTime=1
  Delay{3..7,10..11} (7 alike) : Delay  DelayLength=1  InitialCondition=0
  Delay2 : Delay  DelayLength=3  InitialCondition=0  SampleTime=1
  Delay8 : Delay  DelayLength=3  InitialCondition=0
  Delay9 : Delay  DelayLength=3  InitialCondition=0
  Detect Rise Positive : simulink/Logic and Bit Operations/Detect Rise Positive  vinit=0  OutDataTypeStr=boolean
  Detect Rise Positive5 : hdlsllib/Logic and Bit Operations/Detect Rise Positive  vinit=0  OutDataTypeStr=boolean
  Ground3 : Ground
  Ground4 : Ground
  HDL Counter3 : hdlsllib/Sources/HDL Counter  CountType=Count limited  CountInit=0  CountStep=1  CountMax=2  CountFromType=Initial value  CountFrom=0  CountResetPort=on  CountLoadPort=off  CountEnbPort=on  CountDirPort=off  CountHitOutputPort=on  CountDataType=Unsigned  CountWordLen=2  CountFracLen=0  CountSampTime=1
  HDL Counter4 : hdlsllib/Sources/HDL Counter  CountType=Count limited  CountInit=0  CountStep=1  CountMax=2  CountFromType=Initial value  CountFrom=0  CountResetPort=on  CountLoadPort=off  CountEnbPort=on  CountDirPort=off  CountHitOutputPort=on  CountDataType=Unsigned  CountWordLen=2  CountFracLen=0  CountSampTime=1
  HDL Counter5 : hdlsllib/Sources/HDL Counter  CountType=Count limited  CountInit=0  CountStep=1  CountMax=1  CountFromType=Initial value  CountFrom=0  CountResetPort=off  CountLoadPort=off  CountEnbPort=on  CountDirPort=off  CountHitOutputPort=off  CountDataType=Unsigned  CountWordLen=1  CountFracLen=0  CountSampTime=1
  HDL FIFO : hdlsllib/HDL RAMs/HDL FIFO  fifo_size=792  mode=Classic  ratio=1  push_msg=Warning  pop_msg=Ignore  show_empty=on  show_full=on  show_num=on  LabelModeActiveChoice_Mode=Classic  rst_port=off
  Logical Operator : Logic  Operator=OR  AllPortsSameDT=off  OutDataTypeStr=boolean
  Logical Operator8 : Logic  Operator=OR  AllPortsSameDT=off  OutDataTypeStr=boolean
  Logical Operator9 : Logic  Operator=OR  AllPortsSameDT=off  OutDataTypeStr=boolean
  Multiport Switch{1..5} (5 alike) : MultiPortSwitch  Inputs=2  DiagnosticForDefault=None  SaturateOnIntegerOverflow=off  InputSameDT=off
  Sample Control Bus Selector : whdlutilities/Sample Control Bus Selector  OutputSignals=start,end,valid
  Sample Control Bus Selector1 : whdlutilities/Sample Control Bus Selector  OutputSignals=start,end,valid
  Simple Dual Port RAM : hdlsllib/HDL RAMs/Simple Dual Port RAM  ram_size=2
  Switch5 : Switch  Criteria=u2 ~= 0  SaturateOnIntegerOverflow=off  InputSameDT=off
  Switch6 : Switch  Criteria=u2 ~= 0  SaturateOnIntegerOverflow=off  InputSameDT=off
  Terminator{,1..3} (4 alike) : Terminator
  port1_syn : Outport  VectorParamsAs1DForOutWhenUnconnected=off
  port2_syn : Outport  Port=2  VectorParamsAs1DForOutWhenUnconnected=off
  valid_syn : Outport  Port=3  OutDataTypeStr=boolean  VectorParamsAs1DForOutWhenUnconnected=off
  start_syn : Outport  Port=4  OutDataTypeStr=boolean  VectorParamsAs1DForOutWhenUnconnected=off
  wires:
  port1_ctrl/1 -> Sample Control Bus Selector/1
  port2_ctrl/1 -> Sample Control Bus Selector1/1
  Sample Control Bus Selector/1 -> Logical Operator/1
  Sample Control Bus Selector1/1 -> Logical Operator/2
  Sample Control Bus Selector/2 -> Logical Operator8/1
  Delay7/1 -> HDL Counter4/1
  HDL Counter4/2 -> Delay7/1
  Compare To Constant10/1 -> Detect Rise Positive5/1
  Logical Operator8/1 -> HDL Counter3/2
  HDL Counter3/2 -> Logical Operator9/2, Delay6/1
  HDL Counter3/1 -> Terminator2/1
  Delay6/1 -> HDL Counter3/1
  Logical Operator/1 -> HDL Counter4/2
  Detect Rise Positive5/1 -> Logical Operator9/1
  HDL Counter4/1 -> Compare To Constant10/1
  HDL Counter5/1 -> Data Type Conversion1/1
  Logical Operator9/1 -> HDL Counter5/1, Simple Dual Port RAM/3
  Bit Concat/1 -> Simple Dual Port RAM/1
  Constant3/1 -> Simple Dual Port RAM/4, Simple Dual Port RAM/2
  Data Type Conversion1/1 -> Delay3/1
  Sample Control Bus Selector1/2 -> Logical Operator8/2
  Simple Dual Port RAM/1 -> [number]
  port1/1 -> Delay1/1
  port2/1 -> Delay2/1
  Multiport Switch1/1 -> HDL FIFO/2
  HDL FIFO/1 -> Multiport Switch5/3, Multiport Switch4/2
  HDL FIFO/3 -> Terminator/1
  Multiport Switch3/1 -> HDL FIFO/1
  Multiport Switch2/1 -> HDL FIFO/3, Delay11/1
  [number] -> Multiport Switch2/1, Multiport Switch1/1, Multiport Switch3/1
  Sample Control Bus Selector/3 -> Delay9/1, Bit Concat/2
  Sample Control Bus Selector1/3 -> Delay8/1, Bit Concat/1
  Delay2/1 -> [P2], Multiport Switch3/3
  Delay3/1 -> [number_valid]
  Delay8/1 -> Multiport Switch2/2, Multiport Switch1/3
  Delay9/1 -> Multiport Switch2/3, Multiport Switch1/2
  HDL FIFO/2 -> Terminator1/1
  HDL FIFO/4 -> Terminator3/1
  [number] -> Delay4/1
  Delay4/1 -> Multiport Switch5/1, Multiport Switch4/1
  Delay1/1 -> [P1], Multiport Switch3/2
  [P1] -> Delay5/1
  [P2] -> Delay10/1
  Delay10/1 -> Multiport Switch5/2
  Delay5/1 -> Multiport Switch4/3
  Ground4/1 -> Switch6/3
  Switch5/1 -> port1_syn/1  "port1_syn"
  Switch6/1 -> port2_syn/1  "port2_syn"
  Ground3/1 -> Switch5/3
  Multiport Switch4/1 -> Switch5/1
  Multiport Switch5/1 -> Switch6/1
  Delay11/1 -> Switch5/2, Switch6/2, Detect Rise Positive/1, valid_syn/1
  Detect Rise Positive/1 -> start_syn/1

== system rx2/process4/decoder/synchronization/data_synchronization7 ==
  port1 : Inport
  port2 : Inport  Port=2
  port1_ctrl : Inport  Port=3  OutDataTypeStr=Bus: samplecontrol
  port2_ctrl : Inport  Port=4  OutDataTypeStr=Bus: samplecontrol
  Bit Concat : hdlsllib/Logic and Bit Operations/Bit Concat  numInputs=2
  Compare To Constant10 : hdlsllib/Logic and Bit Operations/Compare To Constant  relop===  const=1  OutDataTypeStr=boolean
  Constant3 : Constant  OutDataTypeStr=fixdt(0,2,0)
  Data Type Conversion1 : DataTypeConversion  OutDataTypeStr=boolean  SaturateOnIntegerOverflow=off  RndMeth=Floor
  Delay1 : Delay  DelayLength=3  InitialCondition=0  SampleTime=1
  Delay{3..7,10..11} (7 alike) : Delay  DelayLength=1  InitialCondition=0
  Delay2 : Delay  DelayLength=3  InitialCondition=0  SampleTime=1
  Delay8 : Delay  DelayLength=3  InitialCondition=0
  Delay9 : Delay  DelayLength=3  InitialCondition=0
  Detect Rise Positive : simulink/Logic and Bit Operations/Detect Rise Positive  vinit=0  OutDataTypeStr=boolean
  Detect Rise Positive5 : hdlsllib/Logic and Bit Operations/Detect Rise Positive  vinit=0  OutDataTypeStr=boolean
  Ground3 : Ground
  Ground4 : Ground
  HDL Counter3 : hdlsllib/Sources/HDL Counter  CountType=Count limited  CountInit=0  CountStep=1  CountMax=2  CountFromType=Initial value  CountFrom=0  CountResetPort=on  CountLoadPort=off  CountEnbPort=on  CountDirPort=off  CountHitOutputPort=on  CountDataType=Unsigned  CountWordLen=2  CountFracLen=0  CountSampTime=1
  HDL Counter4 : hdlsllib/Sources/HDL Counter  CountType=Count limited  CountInit=0  CountStep=1  CountMax=2  CountFromType=Initial value  CountFrom=0  CountResetPort=on  CountLoadPort=off  CountEnbPort=on  CountDirPort=off  CountHitOutputPort=on  CountDataType=Unsigned  CountWordLen=2  CountFracLen=0  CountSampTime=1
  HDL Counter5 : hdlsllib/Sources/HDL Counter  CountType=Count limited  CountInit=0  CountStep=1  CountMax=1  CountFromType=Initial value  CountFrom=0  CountResetPort=off  CountLoadPort=off  CountEnbPort=on  CountDirPort=off  CountHitOutputPort=off  CountDataType=Unsigned  CountWordLen=1  CountFracLen=0  CountSampTime=1
  HDL FIFO : hdlsllib/HDL RAMs/HDL FIFO  fifo_size=792  mode=Classic  ratio=1  push_msg=Warning  pop_msg=Ignore  show_empty=on  show_full=on  show_num=on  LabelModeActiveChoice_Mode=Classic  rst_port=off
  Logical Operator : Logic  Operator=OR  AllPortsSameDT=off  OutDataTypeStr=boolean
  Logical Operator8 : Logic  Operator=OR  AllPortsSameDT=off  OutDataTypeStr=boolean
  Logical Operator9 : Logic  Operator=OR  AllPortsSameDT=off  OutDataTypeStr=boolean
  Multiport Switch{1..5} (5 alike) : MultiPortSwitch  Inputs=2  DiagnosticForDefault=None  SaturateOnIntegerOverflow=off  InputSameDT=off
  Sample Control Bus Selector : whdlutilities/Sample Control Bus Selector  OutputSignals=start,end,valid
  Sample Control Bus Selector1 : whdlutilities/Sample Control Bus Selector  OutputSignals=start,end,valid
  Simple Dual Port RAM : hdlsllib/HDL RAMs/Simple Dual Port RAM  ram_size=2
  Switch5 : Switch  Criteria=u2 ~= 0  SaturateOnIntegerOverflow=off  InputSameDT=off
  Switch6 : Switch  Criteria=u2 ~= 0  SaturateOnIntegerOverflow=off  InputSameDT=off
  Terminator{,1..3} (4 alike) : Terminator
  port1_syn : Outport  VectorParamsAs1DForOutWhenUnconnected=off
  port2_syn : Outport  Port=2  VectorParamsAs1DForOutWhenUnconnected=off
  valid_syn : Outport  Port=3  OutDataTypeStr=boolean  VectorParamsAs1DForOutWhenUnconnected=off
  start_syn : Outport  Port=4  OutDataTypeStr=boolean  VectorParamsAs1DForOutWhenUnconnected=off
  wires:
  port1_ctrl/1 -> Sample Control Bus Selector/1
  port2_ctrl/1 -> Sample Control Bus Selector1/1
  Sample Control Bus Selector/1 -> Logical Operator/1
  Sample Control Bus Selector1/1 -> Logical Operator/2
  Sample Control Bus Selector/2 -> Logical Operator8/1
  Delay7/1 -> HDL Counter4/1
  HDL Counter4/2 -> Delay7/1
  Compare To Constant10/1 -> Detect Rise Positive5/1
  Logical Operator8/1 -> HDL Counter3/2
  HDL Counter3/2 -> Logical Operator9/2, Delay6/1
  HDL Counter3/1 -> Terminator2/1
  Delay6/1 -> HDL Counter3/1
  Logical Operator/1 -> HDL Counter4/2
  Detect Rise Positive5/1 -> Logical Operator9/1
  HDL Counter4/1 -> Compare To Constant10/1
  HDL Counter5/1 -> Data Type Conversion1/1
  Logical Operator9/1 -> HDL Counter5/1, Simple Dual Port RAM/3
  Bit Concat/1 -> Simple Dual Port RAM/1
  Constant3/1 -> Simple Dual Port RAM/4, Simple Dual Port RAM/2
  Data Type Conversion1/1 -> Delay3/1
  Sample Control Bus Selector1/2 -> Logical Operator8/2
  Simple Dual Port RAM/1 -> [number]
  port1/1 -> Delay1/1
  port2/1 -> Delay2/1
  Multiport Switch1/1 -> HDL FIFO/2
  HDL FIFO/1 -> Multiport Switch5/3, Multiport Switch4/2
  HDL FIFO/3 -> Terminator/1
  Multiport Switch3/1 -> HDL FIFO/1
  Multiport Switch2/1 -> HDL FIFO/3, Delay11/1
  [number] -> Multiport Switch2/1, Multiport Switch1/1, Multiport Switch3/1
  Sample Control Bus Selector/3 -> Delay9/1, Bit Concat/2
  Sample Control Bus Selector1/3 -> Delay8/1, Bit Concat/1
  Delay2/1 -> [P2], Multiport Switch3/3
  Delay3/1 -> [number_valid]
  Delay8/1 -> Multiport Switch2/2, Multiport Switch1/3
  Delay9/1 -> Multiport Switch2/3, Multiport Switch1/2
  HDL FIFO/2 -> Terminator1/1
  HDL FIFO/4 -> Terminator3/1
  [number] -> Delay4/1
  Delay4/1 -> Multiport Switch5/1, Multiport Switch4/1
  Delay1/1 -> [P1], Multiport Switch3/2
  [P1] -> Delay5/1
  [P2] -> Delay10/1
  Delay10/1 -> Multiport Switch5/2
  Delay5/1 -> Multiport Switch4/3
  Ground4/1 -> Switch6/3
  Switch5/1 -> port1_syn/1  "port1_syn"
  Switch6/1 -> port2_syn/1  "port2_syn"
  Ground3/1 -> Switch5/3
  Multiport Switch4/1 -> Switch5/1
  Multiport Switch5/1 -> Switch6/1
  Delay11/1 -> Switch5/2, Switch6/2, Detect Rise Positive/1, valid_syn/1
  Detect Rise Positive/1 -> start_syn/1
